simulink model "DBLOQUES"  (R2013a)
settings: Solver=ode45  StartTime=0.0  StopTime=10.0  RelTol=1e-3
settings Model: Creator=tp.aulas3  LastModifiedBy=mario

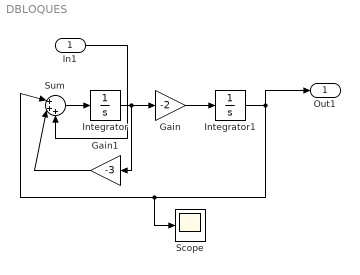
== system DBLOQUES ==
  In1 : Inport
  Gain : Gain  Gain=-2
  Gain1 : Gain  Gain=-3
  Integrator : Integrator
  Integrator1 : Integrator
  Scope : Scope
  Sum : Sum  Inputs=|+++
  Out1 : Outport
  wires:
  Sum/1 -> Integrator/1
  Integrator/1 -> Gain/1, Gain1/1
  Gain/1 -> Integrator1/1
  Integrator1/1 -> Out1/1, Scope/1, Sum/1
  Gain1/1 -> Sum/2
  In1/1 -> Sum/3
